simulink model "PiSimulink_RPi"  (R2020b)
settings: Solver=FixedStepDiscrete  StartTime=0.0  StopTime=10  FixedStep=0.01  RelTol=1e-3  EnableMultiTasking=on
libraries: embdlinuxlib x2, simulink x1, raspberrypiCommlib x1
settings Model: Creator=Audesse  LastModifiedBy=cbeal
settings SolverCC: PositivePriorityOrder=on
settings DataIOCC: SaveFormat=Array  ReturnWorkspaceOutputs=off
settings OptimizationCC: DefaultUnderspecifiedDataType=single  EnhancedBackFolding=on  PassReuseOutputArgsAs=Individual arguments  MaxStackSize=64  OptimizeBlockOrder=speed  DifferentSizesBufferReuse=on  OptimizationCustomize=off  EfficientTunableParamExpr=on
settings DebuggingCC: ParameterTunabilityLossMsg=error
settings HardwareCC: ProdBitPerPointer=32  ProdBitPerSizeT=32  ProdBitPerPtrDiffT=32  ProdLargestAtomicInteger=Long  ProdLargestAtomicFloat=Double  ProdWordSize=32  ProdLongLongMode=on  ProdHWDeviceType=ARM Compatible->ARM Cortex
settings SFSimCC: MATLABDynamicMemAlloc=off  CustomCodeUndefinedFunction=UseInterfaceOnly
settings RTWCC: Description=Embedded Coder  SystemTargetFile=ert.tlc  HardwareBoard=Raspberry Pi  TLCOptions="-aInlineSetEventsForThisBaseRateFcn=TLC_FALSE -aSuppressMultiTaskScheduler=TLC_FALSE  -aRateBasedStepFcn=0"  TemplateMakefile=ert_default_tmf  GenerateReport=on  Toolchain=GNU GCC Raspberry Pi  BuildConfiguration=Faster Runs  IncludeHyperlinkInReport=on  LaunchReport=on  GenerateTraceInfo=on  GenerateTraceReport=on  GenerateTraceReportSl=on  GenerateTraceReportSf=on  GenerateTraceReportEml=on
settings CodeAppCC: ForceParamTrailComments=on  IgnoreCustomStorageClasses=off  OperatorAnnotations=on  SimulinkDataObjDesc=on  SFDataObjDesc=on  InsertBlockDesc=on
settings ERTTargetCC: MatFileLogging=on  SupportVariableSizeSignals=on

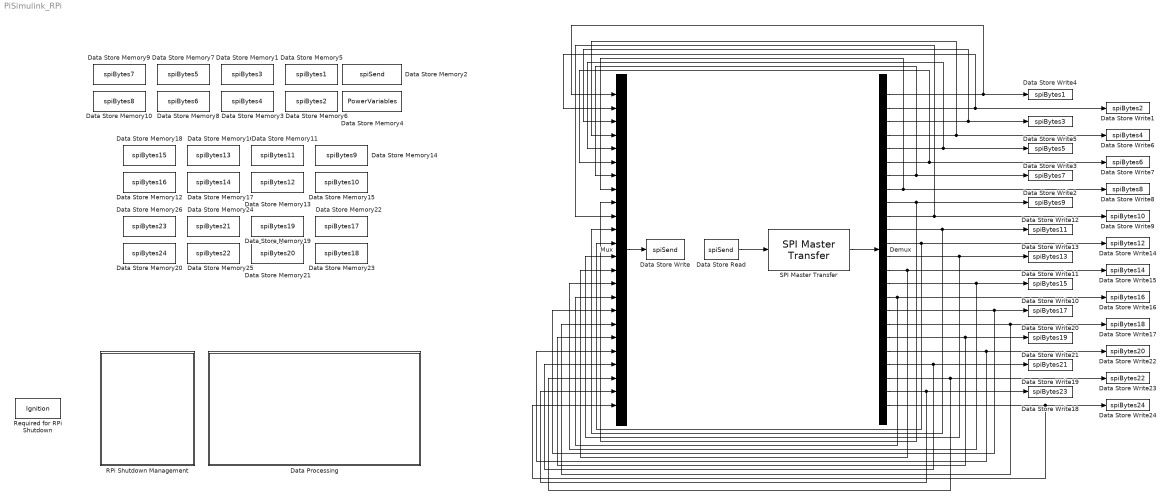
== system PiSimulink_RPi ==
  Data Processing : Subsystem
  Data Store Memory1 : DataStoreMemory  DataStoreName=spiBytes3  ReadBeforeWriteMsg=warning  WriteAfterWriteMsg=warning  WriteAfterReadMsg=warning  InitialValue=[255 255 255 255 255 255 255 255]  ShowAdditionalParam=off  OutDataTypeStr=uint8
  Data Store Memory10 : DataStoreMemory  DataStoreName=spiBytes8  ReadBeforeWriteMsg=warning  WriteAfterWriteMsg=warning  WriteAfterReadMsg=warning  InitialValue=[255 255 255 255 255 255 255 255]  ShowAdditionalParam=off  OutDataTypeStr=uint8
  Data Store Memory11 : DataStoreMemory  DataStoreName=spiBytes11  ReadBeforeWriteMsg=warning  WriteAfterWriteMsg=warning  WriteAfterReadMsg=warning  InitialValue=[255 255 255 255 255 255 255 255]  ShowAdditionalParam=off  OutDataTypeStr=uint8
  Data Store Memory12 : DataStoreMemory  DataStoreName=spiBytes16  ReadBeforeWriteMsg=warning  WriteAfterWriteMsg=warning  WriteAfterReadMsg=warning  InitialValue=[255 255 255 255 255 255 255 255]  ShowAdditionalParam=off  OutDataTypeStr=uint8
  Data Store Memory13 : DataStoreMemory  DataStoreName=spiBytes12  ReadBeforeWriteMsg=warning  WriteAfterWriteMsg=warning  WriteAfterReadMsg=warning  InitialValue=[255 255 255 255 255 255 255 255]  ShowAdditionalParam=off  OutDataTypeStr=uint8
  Data Store Memory14 : DataStoreMemory  DataStoreName=spiBytes9  ReadBeforeWriteMsg=warning  WriteAfterWriteMsg=warning  WriteAfterReadMsg=warning  InitialValue=[255 255 255 255 255 255 255 255]  ShowAdditionalParam=off  OutDataTypeStr=uint8
  Data Store Memory15 : DataStoreMemory  DataStoreName=spiBytes10  ReadBeforeWriteMsg=warning  WriteAfterWriteMsg=warning  WriteAfterReadMsg=warning  InitialValue=[255 255 255 255 255 255 255 255]  ShowAdditionalParam=off  OutDataTypeStr=uint8
  Data Store Memory16 : DataStoreMemory  DataStoreName=spiBytes13  ReadBeforeWriteMsg=warning  WriteAfterWriteMsg=warning  WriteAfterReadMsg=warning  InitialValue=[255 255 255 255 255 255 255 255]  ShowAdditionalParam=off  OutDataTypeStr=uint8
  Data Store Memory17 : DataStoreMemory  DataStoreName=spiBytes14  ReadBeforeWriteMsg=warning  WriteAfterWriteMsg=warning  WriteAfterReadMsg=warning  InitialValue=[255 255 255 255 255 255 255 255]  ShowAdditionalParam=off  OutDataTypeStr=uint8
  Data Store Memory18 : DataStoreMemory  DataStoreName=spiBytes15  ReadBeforeWriteMsg=warning  WriteAfterWriteMsg=warning  WriteAfterReadMsg=warning  InitialValue=[255 255 255 255 255 255 255 255]  ShowAdditionalParam=off  OutDataTypeStr=uint8
  Data Store Memory19 : DataStoreMemory  DataStoreName=spiBytes19  ReadBeforeWriteMsg=warning  WriteAfterWriteMsg=warning  WriteAfterReadMsg=warning  InitialValue=[255 255 255 255 255 255 255 255]  ShowAdditionalParam=off  OutDataTypeStr=uint8
  Data Store Memory2 : DataStoreMemory  DataStoreName=spiSend  ReadBeforeWriteMsg=warning  WriteAfterWriteMsg=warning  WriteAfterReadMsg=warning  InitialValue=zeros(1,192)  ShowAdditionalParam=off  OutDataTypeStr=uint8
  Data Store Memory20 : DataStoreMemory  DataStoreName=spiBytes24  ReadBeforeWriteMsg=warning  WriteAfterWriteMsg=warning  WriteAfterReadMsg=warning  InitialValue=[255 255 255 255 255 255 255 255]  ShowAdditionalParam=off  OutDataTypeStr=uint8
  Data Store Memory21 : DataStoreMemory  DataStoreName=spiBytes20  ReadBeforeWriteMsg=warning  WriteAfterWriteMsg=warning  WriteAfterReadMsg=warning  InitialValue=[255 255 255 255 255 255 255 255]  ShowAdditionalParam=off  OutDataTypeStr=uint8
  Data Store Memory22 : DataStoreMemory  DataStoreName=spiBytes17  ReadBeforeWriteMsg=warning  WriteAfterWriteMsg=warning  WriteAfterReadMsg=warning  InitialValue=[255 255 255 255 255 255 255 255]  ShowAdditionalParam=off  OutDataTypeStr=uint8
  Data Store Memory23 : DataStoreMemory  DataStoreName=spiBytes18  ReadBeforeWriteMsg=warning  WriteAfterWriteMsg=warning  WriteAfterReadMsg=warning  InitialValue=[255 255 255 255 255 255 255 255]  ShowAdditionalParam=off  OutDataTypeStr=uint8
  Data Store Memory24 : DataStoreMemory  DataStoreName=spiBytes21  ReadBeforeWriteMsg=warning  WriteAfterWriteMsg=warning  WriteAfterReadMsg=warning  InitialValue=[255 255 255 255 255 255 255 255]  ShowAdditionalParam=off  OutDataTypeStr=uint8
  Data Store Memory25 : DataStoreMemory  DataStoreName=spiBytes22  ReadBeforeWriteMsg=warning  WriteAfterWriteMsg=warning  WriteAfterReadMsg=warning  InitialValue=[255 255 255 255 255 255 255 255]  ShowAdditionalParam=off  OutDataTypeStr=uint8
  Data Store Memory26 : DataStoreMemory  DataStoreName=spiBytes23  ReadBeforeWriteMsg=warning  WriteAfterWriteMsg=warning  WriteAfterReadMsg=warning  InitialValue=[255 255 255 255 255 255 255 255]  ShowAdditionalParam=off  OutDataTypeStr=uint8
  Data Store Memory3 : DataStoreMemory  DataStoreName=spiBytes4  ReadBeforeWriteMsg=warning  WriteAfterWriteMsg=warning  WriteAfterReadMsg=warning  InitialValue=[255 255 255 255 255 255 255 255]  ShowAdditionalParam=off  OutDataTypeStr=uint8
  Data Store Memory4 : DataStoreMemory  DataStoreName=PowerVariables  ReadBeforeWriteMsg=warning  WriteAfterWriteMsg=warning  WriteAfterReadMsg=warning  InitialValue=[0 0 0 0 0 0 0 0]  ShowAdditionalParam=off  OutDataTypeStr=uint8
  Data Store Memory5 : DataStoreMemory  DataStoreName=spiBytes1  ReadBeforeWriteMsg=warning  WriteAfterWriteMsg=warning  WriteAfterReadMsg=warning  InitialValue=[255 255 255 255 255 255 255 255]  ShowAdditionalParam=off  OutDataTypeStr=uint8
  Data Store Memory6 : DataStoreMemory  DataStoreName=spiBytes2  ReadBeforeWriteMsg=warning  WriteAfterWriteMsg=warning  WriteAfterReadMsg=warning  InitialValue=[255 255 255 255 255 255 255 255]  ShowAdditionalParam=off  OutDataTypeStr=uint8
  Data Store Memory7 : DataStoreMemory  DataStoreName=spiBytes5  ReadBeforeWriteMsg=warning  WriteAfterWriteMsg=warning  WriteAfterReadMsg=warning  InitialValue=[255 255 255 255 255 255 255 255]  ShowAdditionalParam=off  OutDataTypeStr=uint8
  Data Store Memory8 : DataStoreMemory  DataStoreName=spiBytes6  ReadBeforeWriteMsg=warning  WriteAfterWriteMsg=warning  WriteAfterReadMsg=warning  InitialValue=[255 255 255 255 255 255 255 255]  ShowAdditionalParam=off  OutDataTypeStr=uint8
  Data Store Memory9 : DataStoreMemory  DataStoreName=spiBytes7  ReadBeforeWriteMsg=warning  WriteAfterWriteMsg=warning  WriteAfterReadMsg=warning  InitialValue=[255 255 255 255 255 255 255 255]  ShowAdditionalParam=off  OutDataTypeStr=uint8
  Data Store Read : DataStoreRead  DataStoreName=spiSend
  Data Store Write : DataStoreWrite  DataStoreName=spiSend
  Data Store Write1 : DataStoreWrite  DataStoreName=spiBytes2
  Data Store Write10 : DataStoreWrite  DataStoreName=spiBytes15
  Data Store Write11 : DataStoreWrite  DataStoreName=spiBytes13
  Data Store Write12 : DataStoreWrite  DataStoreName=spiBytes9
  Data Store Write13 : DataStoreWrite  DataStoreName=spiBytes11
  Data Store Write14 : DataStoreWrite  DataStoreName=spiBytes12
  Data Store Write15 : DataStoreWrite  DataStoreName=spiBytes14
  Data Store Write16 : DataStoreWrite  DataStoreName=spiBytes16
  Data Store Write17 : DataStoreWrite  DataStoreName=spiBytes18
  Data Store Write18 : DataStoreWrite  DataStoreName=spiBytes23
  Data Store Write19 : DataStoreWrite  DataStoreName=spiBytes21
  Data Store Write2 : DataStoreWrite  DataStoreName=spiBytes7
  Data Store Write20 : DataStoreWrite  DataStoreName=spiBytes17
  Data Store Write21 : DataStoreWrite  DataStoreName=spiBytes19
  Data Store Write22 : DataStoreWrite  DataStoreName=spiBytes20
  Data Store Write23 : DataStoreWrite  DataStoreName=spiBytes22
  Data Store Write24 : DataStoreWrite  DataStoreName=spiBytes24
  Data Store Write3 : DataStoreWrite  DataStoreName=spiBytes5
  Data Store Write4 : DataStoreWrite  DataStoreName=spiBytes1
  Data Store Write5 : DataStoreWrite  DataStoreName=spiBytes3
  Data Store Write6 : DataStoreWrite  DataStoreName=spiBytes4
  Data Store Write7 : DataStoreWrite  DataStoreName=spiBytes6
  Data Store Write8 : DataStoreWrite  DataStoreName=spiBytes8
  Data Store Write9 : DataStoreWrite  DataStoreName=spiBytes10
  Demux : Demux  Outputs=24
  Mux : Mux  Inputs=24
  RPi Shutdown Management : Subsystem
  Required for RPi Shutdown : DataStoreMemory  DataStoreName=Ignition  ReadBeforeWriteMsg=warning  WriteAfterWriteMsg=warning  WriteAfterReadMsg=warning  ShowAdditionalParam=off  OutDataTypeStr=uint8
  SPI Master Transfer : raspberrypiCommlib/SPI Master Transfer  BoardProperty=Pi 4 Model B  SPIModule=SPI1  Mode=Master  BusSpeed=1000000  Pin=SPI0_CE0  FirstBitToTransfer=Most significant bit (MSB)  ClockMode=2  BlockFunction=Transfer  RegisterAddress=0  OutputDataType=int8  OutputDataLength=1  SSPin=CS0
      settings: SourceProductBaseCode=RASPPI
  wires:
  Data Store Read/1 -> SPI Master Transfer/1
  SPI Master Transfer/1 -> Demux/1
  Mux/1 -> Data Store Write/1
  Demux/2 -> Mux/2, Data Store Write1/1
  Demux/7 -> Mux/7, Data Store Write2/1
  Demux/8 -> Mux/8, Data Store Write8/1
  Demux/1 -> Mux/1, Data Store Write4/1
  Demux/5 -> Mux/5, Data Store Write3/1
  Demux/4 -> Mux/4, Data Store Write6/1
  Demux/6 -> Mux/6, Data Store Write7/1
  Demux/3 -> Mux/3, Data Store Write5/1
  Demux/13 -> Mux/13, Data Store Write11/1
  Demux/11 -> Mux/11, Data Store Write13/1
  Demux/14 -> Mux/14, Data Store Write15/1
  Demux/15 -> Mux/15, Data Store Write10/1
  Demux/12 -> Mux/12, Data Store Write14/1
  Demux/10 -> Mux/10, Data Store Write9/1
  Demux/9 -> Mux/9, Data Store Write12/1
  Demux/16 -> Mux/16, Data Store Write16/1
  Demux/21 -> Mux/21, Data Store Write19/1
  Demux/19 -> Mux/19, Data Store Write21/1
  Demux/22 -> Mux/22, Data Store Write23/1
  Demux/20 -> Mux/20, Data Store Write22/1
  Demux/18 -> Mux/18, Data Store Write17/1
  Demux/17 -> Mux/17, Data Store Write20/1
  Demux/24 -> Mux/24, Data Store Write24/1
  Demux/23 -> Mux/23, Data Store Write18/1

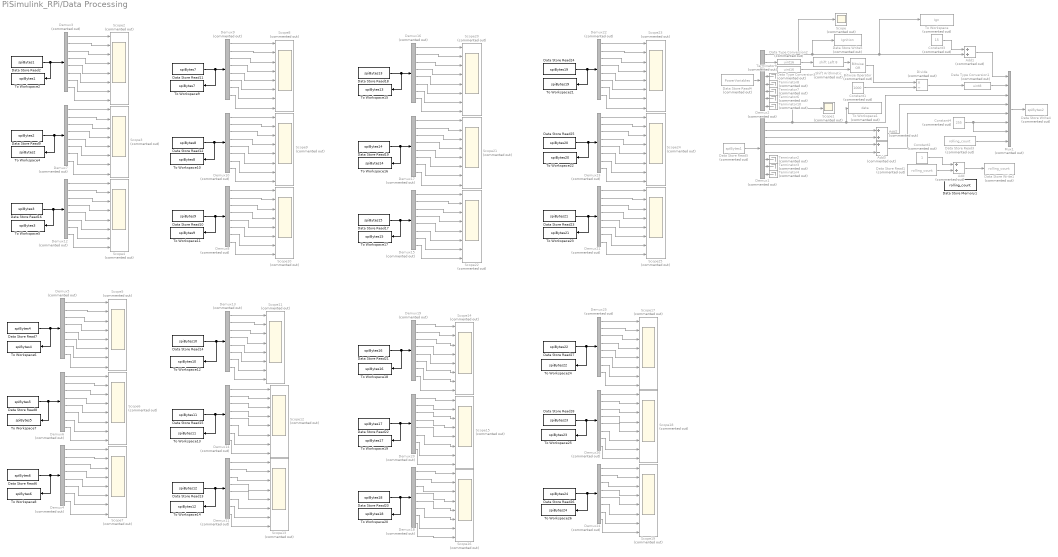
== system PiSimulink_RPi/Data Processing ==
  Add : Sum  Commented=on
  Add1 : Sum  Commented=on
  Add2 : Sum  Commented=on
  Add3 : Sum  Commented=on  Inputs=+-
  Bitwise Operator : simulink/Logic and Bit Operations/Bitwise Operator  Commented=on  logicop=OR  UseBitMask=off  NumInputPorts=2  BitMask=bin2dec('11011001')  BitMaskRealWorld=Stored Integer
  Constant1 : Constant  Commented=on  Value=1000  OutDataTypeStr=uint16
  Constant2 : Constant  Commented=on  OutDataTypeStr=uint8
  Constant3 : Constant  Commented=on  Value=15  OutDataTypeStr=uint8
  Constant4 : Constant  Commented=on  Value=255  OutDataTypeStr=uint8
  Data Store Memory1 : DataStoreMemory  DataStoreName=rolling_count  ReadBeforeWriteMsg=warning  WriteAfterWriteMsg=warning  WriteAfterReadMsg=warning  ShowAdditionalParam=off  OutDataTypeStr=uint8
  Data Store Read1 : DataStoreRead  Commented=on  DataStoreName=rolling_count
  Data Store Read10 : DataStoreRead  DataStoreName=spiBytes9
  Data Store Read11 : DataStoreRead  DataStoreName=spiBytes7
  Data Store Read12 : DataStoreRead  DataStoreName=spiBytes8
  Data Store Read13 : DataStoreRead  DataStoreName=spiBytes12
  Data Store Read14 : DataStoreRead  DataStoreName=spiBytes10
  Data Store Read15 : DataStoreRead  DataStoreName=spiBytes11
  Data Store Read16 : DataStoreRead  DataStoreName=spiBytes3
  Data Store Read17 : DataStoreRead  DataStoreName=spiBytes15
  Data Store Read18 : DataStoreRead  DataStoreName=spiBytes13
  Data Store Read19 : DataStoreRead  DataStoreName=spiBytes14
  Data Store Read2 : DataStoreRead  DataStoreName=spiBytes1
  Data Store Read20 : DataStoreRead  DataStoreName=spiBytes18
  Data Store Read21 : DataStoreRead  DataStoreName=spiBytes16
  Data Store Read22 : DataStoreRead  DataStoreName=spiBytes17
  Data Store Read23 : DataStoreRead  DataStoreName=spiBytes21
  Data Store Read24 : DataStoreRead  DataStoreName=spiBytes19
  Data Store Read25 : DataStoreRead  DataStoreName=spiBytes20
  Data Store Read26 : DataStoreRead  DataStoreName=spiBytes24
  Data Store Read27 : DataStoreRead  DataStoreName=spiBytes22
  Data Store Read28 : DataStoreRead  DataStoreName=spiBytes23
  Data Store Read3 : DataStoreRead  Commented=on  DataStoreName=rolling_count
  Data Store Read4 : DataStoreRead  Commented=on  DataStoreName=PowerVariables
  Data Store Read5 : DataStoreRead  Commented=on  DataStoreName=spiBytes1
  Data Store Read6 : DataStoreRead  DataStoreName=spiBytes6
  Data Store Read7 : DataStoreRead  DataStoreName=spiBytes4
  Data Store Read8 : DataStoreRead  DataStoreName=spiBytes5
  Data Store Read9 : DataStoreRead  DataStoreName=spiBytes2
  Data Store Write1 : DataStoreWrite  Commented=on  DataStoreName=rolling_count
  Data Store Write4 : DataStoreWrite  Commented=on  DataStoreName=spiBytes2
  Data Store Write5 : DataStoreWrite  Commented=on  DataStoreName=Ignition
  Data Type Conversion1 : DataTypeConversion  Commented=on  OutDataTypeStr=uint8
  Data Type Conversion2 : DataTypeConversion  Commented=on  OutDataTypeStr=uint16
  Data Type Conversion3 : DataTypeConversion  Commented=on  OutDataTypeStr=uint16
  Demux{1..26} (26 alike) : Demux  Commented=on  Outputs=8
  Divide : Product  Commented=on  Inputs=*/  OutDataTypeStr=uint16
  Mux1 : Mux  Commented=on  Inputs=8
  Scope : Scope  Commented=on
  Scope1 : Scope  Commented=on
  Scope{2..25} (24 alike) : Scope  Commented=on  NumInputPorts=8
  Shift Arithmetic : ArithShift  Commented=on  BitShiftNumber=8  BitShiftDirection=Left
  Terminator{2..4,6..10} (8 alike) : Terminator  Commented=on
  To Workspace : ToWorkspace  Commented=on  VariableName=Ign  SampleTime=-1
      settings: Save2DSignal=2-D array (concatenate along first dimension)
  To Workspace1 : ToWorkspace  Commented=on  VariableName=data  SampleTime=-1
      settings: Save2DSignal=2-D array (concatenate along first dimension)
  To Workspace10 : ToWorkspace  VariableName=spiBytes8  SampleTime=-1
      settings: Save2DSignal=2-D array (concatenate along first dimension)
  To Workspace11 : ToWorkspace  VariableName=spiBytes9  SampleTime=-1
      settings: Save2DSignal=2-D array (concatenate along first dimension)
  To Workspace12 : ToWorkspace  VariableName=spiBytes10  SampleTime=-1
      settings: Save2DSignal=2-D array (concatenate along first dimension)
  To Workspace13 : ToWorkspace  VariableName=spiBytes11  SampleTime=-1
      settings: Save2DSignal=2-D array (concatenate along first dimension)
  To Workspace14 : ToWorkspace  VariableName=spiBytes12  SampleTime=-1
      settings: Save2DSignal=2-D array (concatenate along first dimension)
  To Workspace15 : ToWorkspace  VariableName=spiBytes13  SampleTime=-1
      settings: Save2DSignal=2-D array (concatenate along first dimension)
  To Workspace16 : ToWorkspace  VariableName=spiBytes14  SampleTime=-1
      settings: Save2DSignal=2-D array (concatenate along first dimension)
  To Workspace17 : ToWorkspace  VariableName=spiBytes15  SampleTime=-1
      settings: Save2DSignal=2-D array (concatenate along first dimension)
  To Workspace18 : ToWorkspace  VariableName=spiBytes16  SampleTime=-1
      settings: Save2DSignal=2-D array (concatenate along first dimension)
  To Workspace19 : ToWorkspace  VariableName=spiBytes17  SampleTime=-1
      settings: Save2DSignal=2-D array (concatenate along first dimension)
  To Workspace2 : ToWorkspace  VariableName=spiBytes1  SampleTime=-1
      settings: Save2DSignal=2-D array (concatenate along first dimension)
  To Workspace20 : ToWorkspace  VariableName=spiBytes18  SampleTime=-1
      settings: Save2DSignal=2-D array (concatenate along first dimension)
  To Workspace21 : ToWorkspace  VariableName=spiBytes19  SampleTime=-1
      settings: Save2DSignal=2-D array (concatenate along first dimension)
  To Workspace22 : ToWorkspace  VariableName=spiBytes20  SampleTime=-1
      settings: Save2DSignal=2-D array (concatenate along first dimension)
  To Workspace23 : ToWorkspace  VariableName=spiBytes21  SampleTime=-1
      settings: Save2DSignal=2-D array (concatenate along first dimension)
  To Workspace24 : ToWorkspace  VariableName=spiBytes22  SampleTime=-1
      settings: Save2DSignal=2-D array (concatenate along first dimension)
  To Workspace25 : ToWorkspace  VariableName=spiBytes23  SampleTime=-1
      settings: Save2DSignal=2-D array (concatenate along first dimension)
  To Workspace26 : ToWorkspace  VariableName=spiBytes24  SampleTime=-1
      settings: Save2DSignal=2-D array (concatenate along first dimension)
  To Workspace4 : ToWorkspace  VariableName=spiBytes2  SampleTime=-1
      settings: Save2DSignal=2-D array (concatenate along first dimension)
  To Workspace5 : ToWorkspace  VariableName=spiBytes3  SampleTime=-1
      settings: Save2DSignal=2-D array (concatenate along first dimension)
  To Workspace6 : ToWorkspace  VariableName=spiBytes4  SampleTime=-1
      settings: Save2DSignal=2-D array (concatenate along first dimension)
  To Workspace7 : ToWorkspace  VariableName=spiBytes5  SampleTime=-1
      settings: Save2DSignal=2-D array (concatenate along first dimension)
  To Workspace8 : ToWorkspace  VariableName=spiBytes6  SampleTime=-1
      settings: Save2DSignal=2-D array (concatenate along first dimension)
  To Workspace9 : ToWorkspace  VariableName=spiBytes7  SampleTime=-1
      settings: Save2DSignal=2-D array (concatenate along first dimension)
  wires:
  Constant4/1 -> Mux1/7, Mux1/6
  Constant2/1 -> Add/1
  Demux1/2 -> Add2/1
  Add/1 -> Data Store Write1/1
  Data Store Read1/1 -> Add/2
  Add1/1 -> Mux1/1
  Demux1/4 -> Add3/1
  Data Store Read5/1 -> Demux1/1
  Demux1/7 -> Terminator3/1
  Demux2/8 -> Terminator10/1
  Demux2/4 -> Terminator9/1
  Demux1/6 -> Terminator2/1
  Data Store Read4/1 -> Demux2/1
  Constant1/1 -> Divide/2
  Data Store Read3/1 -> Mux1/8
  Demux2/7 -> Terminator6/1
  Demux1/8 -> Terminator4/1
  Demux2/6 -> Terminator7/1
  Add2/1 -> Mux1/4
  Demux2/5 -> Terminator8/1
  Add3/1 -> Mux1/5
  Bitwise Operator/1 -> Divide/1
  Mux1/1 -> Data Store Write4/1
  Demux1/5 -> Add3/2
  Constant3/1 -> Add1/1
  Shift Arithmetic/1 -> Bitwise Operator/1
  Demux1/3 -> Add2/2
  Demux2/2 -> Data Type Conversion2/1
  Demux2/3 -> Data Type Conversion3/1
  Demux1/1 -> Scope1/1, To Workspace1/1, Mux1/3
  Data Type Conversion1/1 -> Mux1/2
  Divide/1 -> Data Type Conversion1/1
  Data Type Conversion2/1 -> Shift Arithmetic/1
  Data Type Conversion3/1 -> Bitwise Operator/2
  Demux2/1 -> Scope/1, To Workspace/1, Add1/2, Data Store Write5/1
  Data Store Read2/1 -> To Workspace2/1, Demux3/1
  Demux3/1 -> Scope2/1
  Demux3/2 -> Scope2/2
  Demux3/3 -> Scope2/3
  Demux3/4 -> Scope2/4
  Demux3/5 -> Scope2/5
  Demux3/6 -> Scope2/6
  Demux3/7 -> Scope2/7
  Demux3/8 -> Scope2/8
  Demux7/7 -> Scope3/7
  Demux7/3 -> Scope3/3
  Demux7/4 -> Scope3/4
  Demux7/2 -> Scope3/2
  Demux7/8 -> Scope3/8
  Demux7/1 -> Scope3/1
  Data Store Read9/1 -> To Workspace4/1, Demux7/1
  Demux7/5 -> Scope3/5
  Demux7/6 -> Scope3/6
  Demux12/4 -> Scope4/4
  Demux12/3 -> Scope4/3
  Data Store Read16/1 -> To Workspace5/1, Demux12/1
  Demux12/2 -> Scope4/2
  Demux12/1 -> Scope4/1
  Demux12/5 -> Scope4/5
  Demux12/7 -> Scope4/7
  Demux12/8 -> Scope4/8
  Demux12/6 -> Scope4/6
  Demux6/7 -> Scope6/7
  Data Store Read6/1 -> To Workspace8/1, Demux4/1
  Demux6/8 -> Scope6/8
  Demux6/1 -> Scope6/1
  Data Store Read7/1 -> To Workspace6/1, Demux5/1
  Data Store Read8/1 -> To Workspace7/1, Demux6/1
  Demux5/4 -> Scope5/4
  Demux4/4 -> Scope7/4
  Demux4/1 -> Scope7/1
  Demux5/3 -> Scope5/3
  Demux5/2 -> Scope5/2
  Demux5/1 -> Scope5/1
  Demux5/5 -> Scope5/5
  Demux6/6 -> Scope6/6
  Demux4/7 -> Scope7/7
  Demux4/8 -> Scope7/8
  Demux5/6 -> Scope5/6
  Demux6/2 -> Scope6/2
  Demux4/2 -> Scope7/2
  Demux6/5 -> Scope6/5
  Demux4/5 -> Scope7/5
  Demux5/7 -> Scope5/7
  Demux4/6 -> Scope7/6
  Demux5/8 -> Scope5/8
  Demux6/4 -> Scope6/4
  Demux6/3 -> Scope6/3
  Demux4/3 -> Scope7/3
  Demux10/7 -> Scope9/7
  Data Store Read10/1 -> To Workspace11/1, Demux8/1
  Demux10/8 -> Scope9/8
  Demux10/1 -> Scope9/1
  Data Store Read11/1 -> To Workspace9/1, Demux9/1
  Data Store Read12/1 -> To Workspace10/1, Demux10/1
  Demux9/4 -> Scope8/4
  Demux8/4 -> Scope10/4
  Demux8/1 -> Scope10/1
  Demux9/3 -> Scope8/3
  Demux9/2 -> Scope8/2
  Demux9/1 -> Scope8/1
  Demux9/5 -> Scope8/5
  Demux10/6 -> Scope9/6
  Demux8/7 -> Scope10/7
  Demux8/8 -> Scope10/8
  Demux9/6 -> Scope8/6
  Demux10/2 -> Scope9/2
  Demux8/2 -> Scope10/2
  Demux10/5 -> Scope9/5
  Demux8/5 -> Scope10/5
  Demux9/7 -> Scope8/7
  Demux8/6 -> Scope10/6
  Demux9/8 -> Scope8/8
  Demux10/4 -> Scope9/4
  Demux10/3 -> Scope9/3
  Demux8/3 -> Scope10/3
  Demux14/7 -> Scope12/7
  Data Store Read13/1 -> To Workspace14/1, Demux11/1
  Demux14/8 -> Scope12/8
  Demux14/1 -> Scope12/1
  Data Store Read14/1 -> To Workspace12/1, Demux13/1
  Data Store Read15/1 -> To Workspace13/1, Demux14/1
  Demux13/4 -> Scope11/4
  Demux11/4 -> Scope13/4
  Demux11/1 -> Scope13/1
  Demux13/3 -> Scope11/3
  Demux13/2 -> Scope11/2
  Demux13/1 -> Scope11/1
  Demux13/5 -> Scope11/5
  Demux14/6 -> Scope12/6
  Demux11/7 -> Scope13/7
  Demux11/8 -> Scope13/8
  Demux13/6 -> Scope11/6
  Demux14/2 -> Scope12/2
  Demux11/2 -> Scope13/2
  Demux14/5 -> Scope12/5
  Demux11/5 -> Scope13/5
  Demux13/7 -> Scope11/7
  Demux11/6 -> Scope13/6
  Demux13/8 -> Scope11/8
  Demux14/4 -> Scope12/4
  Demux14/3 -> Scope12/3
  Demux11/3 -> Scope13/3
  Demux17/7 -> Scope21/7
  Data Store Read17/1 -> To Workspace17/1, Demux15/1
  Demux17/8 -> Scope21/8
  Demux17/1 -> Scope21/1
  Data Store Read18/1 -> To Workspace15/1, Demux16/1
  Data Store Read19/1 -> To Workspace16/1, Demux17/1
  Demux16/4 -> Scope20/4
  Demux15/4 -> Scope22/4
  Demux15/1 -> Scope22/1
  Demux16/3 -> Scope20/3
  Demux16/2 -> Scope20/2
  Demux16/1 -> Scope20/1
  Demux16/5 -> Scope20/5
  Demux17/6 -> Scope21/6
  Demux15/7 -> Scope22/7
  Demux15/8 -> Scope22/8
  Demux16/6 -> Scope20/6
  Demux17/2 -> Scope21/2
  Demux15/2 -> Scope22/2
  Demux17/5 -> Scope21/5
  Demux15/5 -> Scope22/5
  Demux16/7 -> Scope20/7
  Demux15/6 -> Scope22/6
  Demux16/8 -> Scope20/8
  Demux17/4 -> Scope21/4
  Demux17/3 -> Scope21/3
  Demux15/3 -> Scope22/3
  Demux20/7 -> Scope15/7
  Data Store Read20/1 -> To Workspace20/1, Demux18/1
  Demux20/8 -> Scope15/8
  Demux20/1 -> Scope15/1
  Data Store Read21/1 -> To Workspace18/1, Demux19/1
  Data Store Read22/1 -> To Workspace19/1, Demux20/1
  Demux19/4 -> Scope14/4
  Demux18/4 -> Scope16/4
  Demux18/1 -> Scope16/1
  Demux19/3 -> Scope14/3
  Demux19/2 -> Scope14/2
  Demux19/1 -> Scope14/1
  Demux19/5 -> Scope14/5
  Demux20/6 -> Scope15/6
  Demux18/7 -> Scope16/7
  Demux18/8 -> Scope16/8
  Demux19/6 -> Scope14/6
  Demux20/2 -> Scope15/2
  Demux18/2 -> Scope16/2
  Demux20/5 -> Scope15/5
  Demux18/5 -> Scope16/5
  Demux19/7 -> Scope14/7
  Demux18/6 -> Scope16/6
  Demux19/8 -> Scope14/8
  Demux20/4 -> Scope15/4
  Demux20/3 -> Scope15/3
  Demux18/3 -> Scope16/3
  Demux25/1 -> Scope17/1
  Demux25/5 -> Scope17/5
  Demux24/7 -> Scope19/7
  Demux25/3 -> Scope17/3
  Data Store Read26/1 -> To Workspace26/1, Demux24/1
  Data Store Read27/1 -> To Workspace24/1, Demux25/1
  Demux26/1 -> Scope18/1
  Demux24/1 -> Scope19/1
  Data Store Read28/1 -> To Workspace25/1, Demux26/1
  Demux26/3 -> Scope18/3
  Demux24/3 -> Scope19/3
  Demux26/8 -> Scope18/8
  Demux24/5 -> Scope19/5
  Demux25/4 -> Scope17/4
  Demux26/2 -> Scope18/2
  Demux25/8 -> Scope17/8
  Demux25/7 -> Scope17/7
  Demux24/6 -> Scope19/6
  Demux26/5 -> Scope18/5
  Demux24/2 -> Scope19/2
  Demux21/3 -> Scope25/3
  Demux23/3 -> Scope24/3
  Demux22/8 -> Scope23/8
  Demux23/4 -> Scope24/4
  Demux22/7 -> Scope23/7
  Demux21/6 -> Scope25/6
  Demux21/5 -> Scope25/5
  Demux21/8 -> Scope25/8
  Demux22/2 -> Scope23/2
  Demux22/6 -> Scope23/6
  Demux22/5 -> Scope23/5
  Demux26/7 -> Scope18/7
  Demux21/7 -> Scope25/7
  Demux26/6 -> Scope18/6
  Demux22/1 -> Scope23/1
  Demux23/2 -> Scope24/2
  Demux23/5 -> Scope24/5
  Demux25/6 -> Scope17/6
  Demux21/2 -> Scope25/2
  Demux26/4 -> Scope18/4
  Demux22/3 -> Scope23/3
  Data Store Read23/1 -> To Workspace23/1, Demux21/1
  Demux21/1 -> Scope25/1
  Demux22/4 -> Scope23/4
  Demux24/8 -> Scope19/8
  Demux21/4 -> Scope25/4
  Demux25/2 -> Scope17/2
  Data Store Read25/1 -> To Workspace22/1, Demux23/1
  Data Store Read24/1 -> To Workspace21/1, Demux22/1
  Demux23/8 -> Scope24/8
  Demux24/4 -> Scope19/4
  Demux23/1 -> Scope24/1
  Demux23/6 -> Scope24/6
  Demux23/7 -> Scope24/7

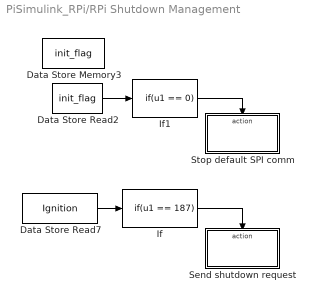
== system PiSimulink_RPi/RPi Shutdown Management ==
  Data Store Memory3 : DataStoreMemory  DataStoreName=init_flag  ReadBeforeWriteMsg=warning  WriteAfterWriteMsg=warning  WriteAfterReadMsg=warning  ShowAdditionalParam=off  OutDataTypeStr=uint8
  Data Store Read2 : DataStoreRead  DataStoreName=init_flag
  Data Store Read7 : DataStoreRead  DataStoreName=Ignition
  If : If  IfExpression=u1 == 187  ShowElse=off
  If1 : If  IfExpression=u1 == 0  ShowElse=off
  Send shutdown request : Subsystem  TreatAsAtomicUnit=on
  Stop default SPI comm : Subsystem  TreatAsAtomicUnit=on
  wires:
  If/1 -> Send shutdown request/Action
  Data Store Read7/1 -> If/1
  If1/1 -> Stop default SPI comm/Action
  Data Store Read2/1 -> If1/1

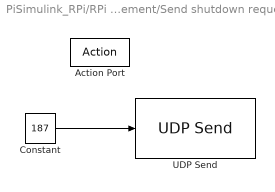
== system PiSimulink_RPi/RPi Shutdown Management/Send shutdown request ==
  Action Port : ActionPort  ActionPortLabel=if(u1 == 187)
  Constant : Constant  Value=187  OutDataTypeStr=uint8
  UDP Send : embdlinuxlib/UDP Send  remoteURL='127.0.0.1'  remotePort=5005  localURL='255.255.255.255'  localPortSource=Automatically determine  localPort=-1  sampletime=-1  blockPlatform=Raspberry Pi  separateLengthPort=0
      settings: SourceProductBaseCode=SC_BEAGLEBONE_BLUE,NVIDIA,RASPPI
  wires:
  Constant/1 -> UDP Send/1

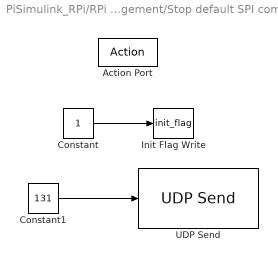
== system PiSimulink_RPi/RPi Shutdown Management/Stop default SPI comm ==
  Action Port : ActionPort  ActionPortLabel=if(u1 == 0)
  Constant : Constant  OutDataTypeStr=uint8
  Constant1 : Constant  Value=131  OutDataTypeStr=uint8
  Init Flag Write : DataStoreWrite  DataStoreName=init_flag
  UDP Send : embdlinuxlib/UDP Send  remoteURL='127.0.0.1'  remotePort=5005  localURL='255.255.255.255'  localPortSource=Automatically determine  localPort=-1  sampletime=-1  blockPlatform=Raspberry Pi  separateLengthPort=0
      settings: SourceProductBaseCode=SC_BEAGLEBONE_BLUE,NVIDIA,RASPPI
  wires:
  Constant/1 -> Init Flag Write/1
  Constant1/1 -> UDP Send/1
